simulink model "ex1subex1"  (R2019a)
settings: Solver=VariableStepAuto  StartTime=0.0  StopTime=10.0  MaxStep=0.003  MinStep=0.001  RelTol=1e-3
settings Model: Creator=toshiba1000  LastModifiedBy=toshiba1000
settings SolverCC: InitialStep=0.002

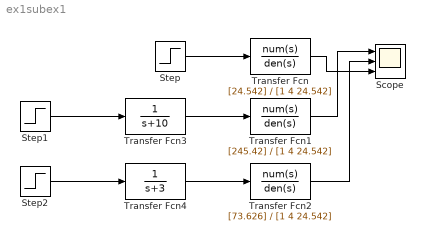
== system ex1subex1 ==
  Scope : Scope  NumInputPorts=3
  Step : Step  SampleTime=0
  Step1 : Step  SampleTime=0
  Step2 : Step  SampleTime=0
  Transfer Fcn : TransferFcn  Numerator=[24.542]  Denominator=[1 4 24.542]
  Transfer Fcn1 : TransferFcn  Numerator=[245.42]  Denominator=[1 4 24.542]
  Transfer Fcn2 : TransferFcn  Numerator=[73.626]  Denominator=[1 4 24.542]
  Transfer Fcn3 : TransferFcn  Denominator=[1 10]
  Transfer Fcn4 : TransferFcn  Denominator=[1 3]
  wires:
  Step/1 -> Transfer Fcn/1
  Transfer Fcn/1 -> Scope/3
  Step1/1 -> Transfer Fcn3/1
  Transfer Fcn1/1 -> Scope/1
  Step2/1 -> Transfer Fcn4/1
  Transfer Fcn2/1 -> Scope/2
  Transfer Fcn3/1 -> Transfer Fcn1/1
  Transfer Fcn4/1 -> Transfer Fcn2/1
